simulink model "pitchonly"  (R2022a)
settings: Solver=VariableStepAuto  StartTime=0.0  StopTime=10.0  RelTol=1e-3
values from neighbouring files (symbols this model uses):
  A_pitch = [0  1; 0  0]    [param.mat]
  B_pitch = [0  0; 0  0.248]    [param.mat]
  C_pitch = [1  0; 0  1]    [param.mat]
  D_pitch = [0  0; 0  0]    [param.mat]
libraries: mpclib x1
settings Model: Creator=marik  LastModifiedBy=marik

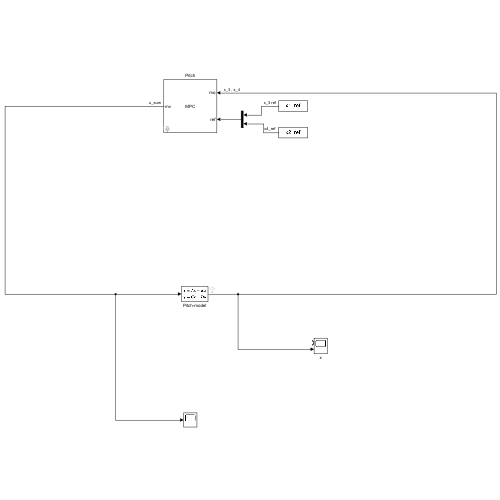
[thumbnail: Simulink's stored preview of the top-level diagram]
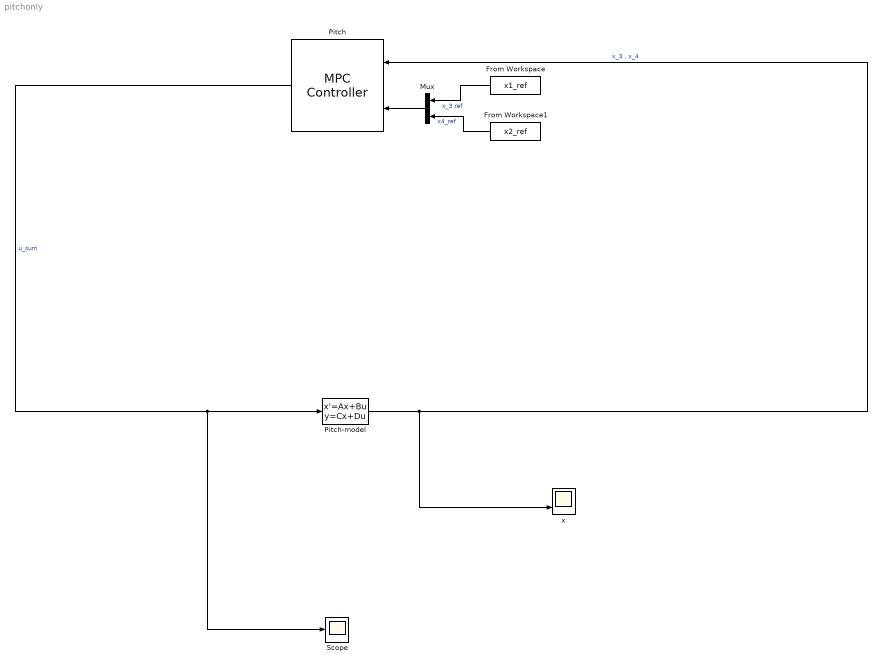
== system pitchonly ==
  From Workspace : FromWorkspace  VariableName=x1_ref  SampleTime=0.1  OutputAfterFinalValue=Holding final value
  From Workspace1 : FromWorkspace  VariableName=x2_ref
  Mux : Mux  Inputs=2
  Pitch : mpclib/MPC Controller  SCDEnableBlockLinearizationSpecification=on  mpcobj=mpcpitch  is_multiple=0  enable_value=0  return_u0=off  updateMPCinCallerWorkspace=on  md_inport=off  mv_inport=off  uref_inport=off  return_cost=off  return_mvseq=off  return_qpstatus=off  return_xseq=off  return_state=off  return_ovseq=off  state_inport=off  umin_inport=off  umax_inport=off  ymin_inport=off  ymax_inport=off  cc_inport=off  ywt_inport=off  uwt_inport=off  duwt_inport=off  rhoeps_inport=off  pm_inport=off  MaximumP=10  HorizonChoice=FixedHorizon  n_ts=0.1  n_p=20  n_mv=2  n_md=0  n_ud=0  n_mo=2  n_uo=0  BlockDataType=double  SampleTimeInherited=off  switch_inport=off
  Pitch-model : StateSpace  A=A_pitch  B=B_pitch  C=C_pitch  D=D_pitch  InitialCondition=0
  Scope : Scope
  x : Scope  NumInputPorts=2
  wires:
  Pitch-model/1 -> x/2, Pitch/1  "x_3 , x_4"
  From Workspace/1 -> Mux/1  "x_3 ref"
  Pitch/1 -> Scope/1, Pitch-model/1  "u_sum"
  From Workspace1/1 -> Mux/2  "x4_ref"
  Mux/1 -> Pitch/2
